simulink model "msg2data"  (R2016a)
settings: Solver=VariableStepAuto  StartTime=0.0  StopTime=inf  RelTol=1e-3
values from neighbouring files (symbols this model uses):
  Tsample = 0.01    [InitCom.m]    (also in init_Kalman.m)
undefined symbols (not defined in the file or in its folder): Ae, Be, Ce, De
libraries: etargetslib x2, dspnetwork x2, utility x1
settings Model: Creator=Florian  LastModifiedBy=Florian

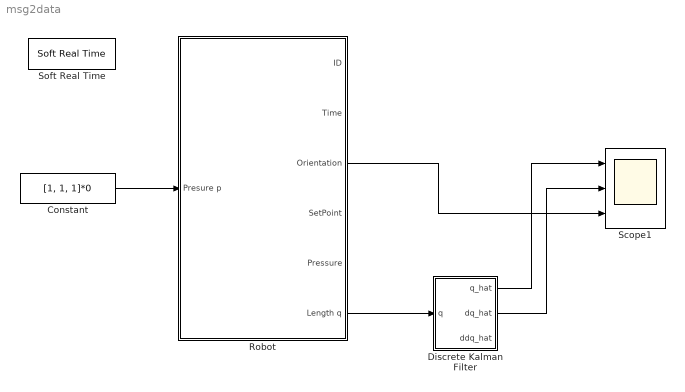
== system msg2data ==
  Constant : Constant  Value=[1, 1, 1]*0
  Discrete Kalman Filter : MATLAB Function  TreatAsAtomicUnit=on  SystemSampleTime=Tsample
  Robot : Subsystem
      mask Display: image('C:\Users\Florian\Documents\Uni\IDP\DVD\Pictures\contibot1seg.JPG');
  Scope1 : Scope  NumInputPorts=3
  Soft Real Time : utility/Soft Real Time  x=1
  wires:
  Discrete Kalman Filter/1(q_hat) -> Scope1/1
  Robot/6(Length q) -> Discrete Kalman Filter/1(q)
  Constant/1 -> Robot/1(Presure p)
  Robot/3(Orientation) -> Scope1/3
  Discrete Kalman Filter/2(dq_hat) -> Scope1/2

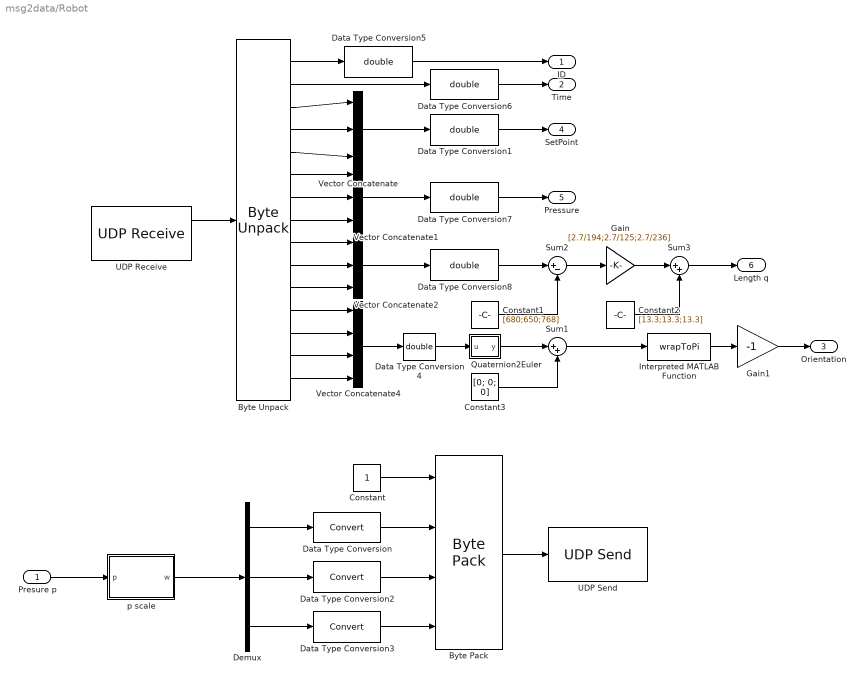
== system msg2data/Robot ==
  Presure p : Inport
  Byte Pack : etargetslib/Byte Pack  datatypes={'uint32', 'uint32', 'uint32', 'uint32'}  byteAlign=1
  Byte Unpack : etargetslib/Byte Unpack  dimensions={[1],[1],[1],[1],[1],[1],[1],[1],[1],[1],[1],[1],[1],[1],[1]}  datatypes={'uint32', 'uint32', 'uint32', 'uint32', 'uint32', 'uint32', 'uint32', 'uint32', 'single', 'single', 'single', 'single', 'single', 'single', 'single'}  byteAlign=1
  Constant : Constant  OutDataTypeStr=uint32
  Constant1 : Constant  Value=[680;650;768]  OutDataTypeStr=uint32
  Constant2 : Constant  Value=[13.3;13.3;13.3]  OutDataTypeStr=uint32
  Constant3 : Constant  Value=[0; 0; 0]  OutDataTypeStr=uint32
  Data Type Conversion : DataTypeConversion
  Data Type Conversion{1,4..8} (6 alike) : DataTypeConversion  OutDataTypeStr=double
  Data Type Conversion2 : DataTypeConversion
  Data Type Conversion3 : DataTypeConversion
  Demux : Demux  Outputs=3
  Gain : Gain  Gain=[2.7/194;2.7/125;2.7/236]
  Gain1 : Gain  Gain=-1
  Interpreted MATLAB Function : MATLABFcn  MATLABFcn=wrapToPi
  Quaternion2Euler : MATLAB Function  TreatAsAtomicUnit=on
  Sum1 : Sum  Inputs=|++
  Sum2 : Sum  Inputs=|+-
  Sum3 : Sum  Inputs=|++
  UDP Receive : dspnetwork/UDP Receive  localURL='0.0.0.0'  localPort=25000  remoteURL='0.0.0.0'  remotePort=-1  recvBufferSize=256  dims=15*4  signalDatatype=uint8  isVarSize=off  showBlockingTime=on  blockingTime=0  sampletime=0.01  blockPlatform=HOST
  UDP Send : dspnetwork/UDP Send  remoteURL='127.0.0.1'  remotePort=12345  localURL='0.0.0.0'  localPortSource=Specify via dialog  localPort=25000  sampletime=-1  blockPlatform=HOST  separateLengthPort=0
  Vector Concatenate : Concatenate  NumInputs=3
  Vector Concatenate1 : Concatenate  NumInputs=3
  Vector Concatenate2 : Concatenate  NumInputs=3
  Vector Concatenate4 : Concatenate  NumInputs=4
  p scale : MATLAB Function  TreatAsAtomicUnit=on
  ID : Outport
  Time : Outport  Port=2
  Orientation : Outport  Port=3
  SetPoint : Outport  Port=4
  Pressure : Outport  Port=5
  Length q : Outport  Port=6
  wires:
  Gain1/1 -> Orientation/1
  Constant3/1 -> Sum1/2
  Sum1/1 -> Interpreted MATLAB Function/1
  Interpreted MATLAB Function/1 -> Gain1/1
  Byte Unpack/9 -> Vector Concatenate2/1
  Constant/1 -> Byte Pack/1
  Vector Concatenate/1 -> Data Type Conversion1/1
  Byte Unpack/6 -> Vector Concatenate1/1
  Sum2/1 -> Gain/1
  Gain/1 -> Sum3/1
  Byte Unpack/4 -> Vector Concatenate/2
  Byte Pack/1 -> UDP Send/1
  Byte Unpack/3 -> Vector Concatenate/1
  Byte Unpack/12 -> Vector Concatenate4/1
  Byte Unpack/5 -> Vector Concatenate/3
  Byte Unpack/13 -> Vector Concatenate4/2
  Constant2/1 -> Sum3/2
  Byte Unpack/14 -> Vector Concatenate4/3
  UDP Receive/1 -> Byte Unpack/1
  Byte Unpack/10 -> Vector Concatenate2/2
  Byte Unpack/7 -> Vector Concatenate1/2
  Byte Unpack/8 -> Vector Concatenate1/3
  Byte Unpack/11 -> Vector Concatenate2/3
  Sum3/1 -> Length q/1
  Byte Unpack/15 -> Vector Concatenate4/4
  Constant1/1 -> Sum2/2
  Quaternion2Euler/1(y) -> Sum1/1
  Vector Concatenate2/1 -> Data Type Conversion8/1
  Data Type Conversion1/1 -> SetPoint/1
  Byte Unpack/1 -> Data Type Conversion5/1
  Data Type Conversion5/1 -> ID/1
  Data Type Conversion6/1 -> Time/1
  Byte Unpack/2 -> Data Type Conversion6/1
  Vector Concatenate1/1 -> Data Type Conversion7/1
  Data Type Conversion7/1 -> Pressure/1
  Data Type Conversion8/1 -> Sum2/1
  Demux/1 -> Data Type Conversion/1
  Demux/2 -> Data Type Conversion2/1
  Presure p/1 -> p scale/1(p)
  Demux/3 -> Data Type Conversion3/1
  Vector Concatenate4/1 -> Data Type Conversion4/1
  Data Type Conversion4/1 -> Quaternion2Euler/1(u)
  Data Type Conversion/1 -> Byte Pack/2
  Data Type Conversion2/1 -> Byte Pack/3
  Data Type Conversion3/1 -> Byte Pack/4
  p scale/1(w) -> Demux/1

== matlab function msg2data/Robot/Quaternion2Euler ==
  data: u input; y output
function y = fcn(u)
%#codegen
u = u / 1000;
y = zeros(3,1);

y(1) = atan2(2*(u(1)*u(2)+u(3)*u(4)),1-2*(u(2)*u(2)+u(3)*u(3)));

if abs(2*(u(1)*u(3)-u(4)*u(2))) > 1
    y(2) = 0;
else
    y(2) = asin(2*(u(1)*u(3)-u(4)*u(2)));
end
y(3) = atan2(2*(u(1)*u(4)+u(2)*u(3)),1-2*(u(3)*u(3)+u(4)*u(4)));

== matlab function msg2data/Discrete Kalman Filter ==
  data: Ae parameter; Be parameter; Ce parameter; De parameter; q input; q_hat output; dq_hat output; ddq_hat output
function [q_hat,dq_hat, ddq_hat] = fcn(Ae,Be,Ce,De,q)
%#codegen
persistent x
if isempty(x)
   x = zeros(3, length(q));%[0;0];
end
 
q_hat = zeros(size(q));
dq_hat = q_hat;
ddq_hat = dq_hat;

for i = 1:length(q)
x_pred = Ae * x(:, i) + Be * q(i);
hat = Ce * x(:, i) + De * q(i);
x(:, i) = x_pred;

y_hat = hat(1);
x_hat = hat(2:4,1);

q_hat(i) = x_hat(1);
dq_hat(i) = x_hat(2);
ddq_hat(i) = x_hat(3);
end

== matlab function msg2data/Robot/p scale ==
  data: p input; w output
function w = fcn(p)
%#codegen

w = (p/1.6 + 1.95) * 500;
